simulink model "AmbientTester"  (R2018b)
settings: Solver=ode1  StartTime=0.0  StopTime=20000  FixedStep=1  RelTol=1e-3
libraries: simulink x1
settings Model: Creator=U375749  LastModifiedBy=U375749

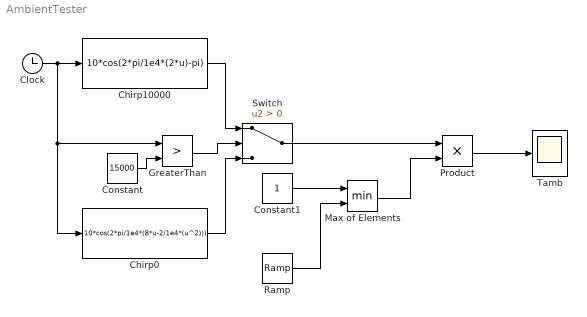
== system AmbientTester ==
  Chirp0 : MATLABFcn  MATLABFcn=10*cos(2*pi/1e4*(8*u-2/1e4*(u^2)))  OutputDimensions=1
  Chirp10000 : MATLABFcn  MATLABFcn=10*cos(2*pi/1e4*(2*u)-pi)  OutputDimensions=1
  Clock : Clock
  Constant : Constant  Value=15000
  Constant1 : Constant
  GreaterThan : RelationalOperator  Operator=>  OutDataTypeStr=boolean  RndMeth=Simplest
  Max of Elements : MinMax  Inputs=2
  Product : Product
  Ramp : simulink/Sources/Ramp  slope=0.75/(10000-6000)  start=6000  InitialOutput=0.25
  Switch : Switch  Criteria=u2 > Threshold
  Tamb : Scope
  wires:
  Switch/1 -> Product/1
  Constant/1 -> GreaterThan/2
  GreaterThan/1 -> Switch/2
  Chirp0/1 -> Switch/3
  Clock/1 -> Chirp0/1, GreaterThan/1, Chirp10000/1
  Chirp10000/1 -> Switch/1
  Product/1 -> Tamb/1
  Ramp/1 -> Max of Elements/2
  Constant1/1 -> Max of Elements/1
  Max of Elements/1 -> Product/2
